simulink model "trap_mf"  (R2016a)
settings: Solver=ode45  StartTime=0.0  StopTime=10.0  RelTol=1e-3
undefined symbols (not defined in the file): fi_1_a, fi_1_b, fi_1_c, fi_1_d
libraries: fuzblock x4
settings Model: Creator=Руслан  LastModifiedBy=Руслан
settings DataIOCC: LimitDataPoints=on  SaveFormat=Array
settings DebuggingCC: AlgebraicLoopMsg=error
settings HardwareCC: ProdBitPerLong=64  ProdLargestAtomicFloat=None  ProdHWDeviceType=Intel->x86-64
settings ModelReferenceCC: PropagateSignalLabelsOutOfModel=off
settings RTWCC: TemplateMakefile=RTW.MSVCBuild  Description=Create Visual C/C++ Solution File for Simulink Coder  GenerateReport=on  RetainRTWFile=on  LaunchReport=on
settings CodeAppCC: ForceParamTrailComments=on  MATLABSourceComments=on
settings GRTTargetCC: TargetLangStandard=C99 (ISO)
settings ConfigComp: CovModelRefEnable=Off

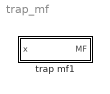
== system trap_mf ==
  trap mf1 : Subsystem  mask{a=fi_1_a, b=fi_1_b, c=fi_1_c, d=fi_1_d}
      mask prompts: a "Left base point a:"; b "Left peak location b:"; c "Right base point c:"; d "Right peak location d:"

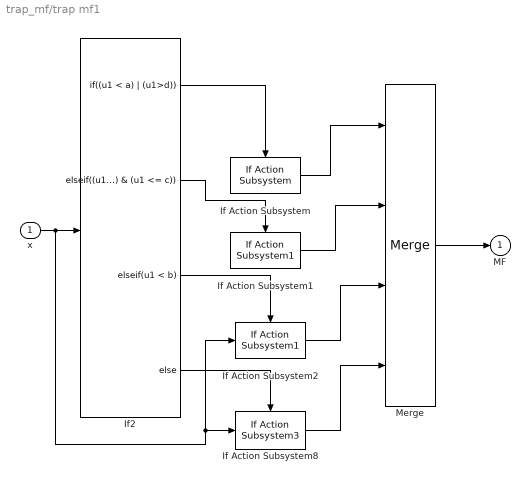
== system trap_mf/trap mf1 ==
  x : Inport
  If Action Subsystem : fuzblock/Membership  Functions/Triangular MF/If Action Subsystem
  If Action Subsystem1 : fuzblock/Membership  Functions/Triangular MF/If Action Subsystem1
  If Action Subsystem2 : fuzblock/Membership  Functions/Trapezoidal MF/If Action Subsystem1
  If Action Subsystem8 : fuzblock/Membership  Functions/Trapezoidal MF/If Action Subsystem3
  If2 : If  IfExpression=(u1 < a) | (u1>d)  ElseIfExpressions=(u1 >= b) & (u1 <= c), u1 < b  ZeroCross=off
  Merge : Merge  Inputs=4
  MF : Outport
  wires:
  If Action Subsystem2/1 -> Merge/3
  If2/3 -> If Action Subsystem2/Action
  If Action Subsystem8/1 -> Merge/4
  If2/4 -> If Action Subsystem8/Action
  If Action Subsystem1/1 -> Merge/2
  If2/2 -> If Action Subsystem1/Action
  If Action Subsystem/1 -> Merge/1
  Merge/1 -> MF/1
  If2/1 -> If Action Subsystem/Action
  x/1 -> If Action Subsystem2/1, If Action Subsystem8/1, If2/1
